simulink model "s0505_rollsensorfusion_CF"  (R2021a)
settings: Solver=FixedStepAuto  StartTime=0.0  StopTime=10.0  RelTol=1e-3  EnableMultiTasking=on
undefined symbols (not defined in the file or in its folder): Ts
libraries: CarMaker4SL x3, dspfdesign x1
settings Model: Creator=jason  LastModifiedBy=jason
settings ModelReferenceCC: ModelReferenceNumInstancesAllowed=Single

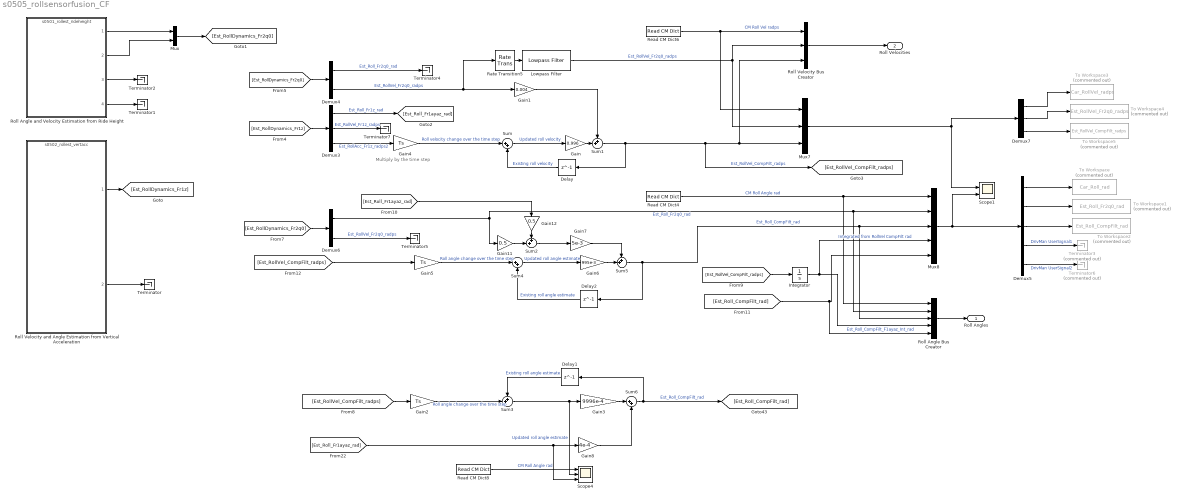
== system s0505_rollsensorfusion_CF ==
  note: Multiply by the time step
  Delay : Delay  DelayLength=1
  Delay1 : Delay  DelayLength=1
  Delay2 : Delay  DelayLength=1
  Demux3 : Demux  Outputs=3
      settings: DisplayOption=none
  Demux4 : Demux  Outputs=2
      settings: DisplayOption=none
  Demux5 : Demux  Outputs=5
      settings: DisplayOption=none
  Demux6 : Demux  Outputs=2
      settings: DisplayOption=none
  Demux7 : Demux  Outputs=3
  Gain : Gain  Gain=0.996
  Gain1 : Gain  Gain=0.004
  Gain11 : Gain  Gain=0.5
  Gain12 : Gain  Gain=0.5
  Gain2 : Gain  Gain=Ts
  Gain3 : Gain  Gain=9996e-4
  Gain4 : Gain  Gain=Ts
  Gain5 : Gain  Gain=Ts
  Gain6 : Gain  Gain=995e-3
  Gain7 : Gain  Gain=5e-3
  Gain8 : Gain  Gain=4e-4
  Integrator : Integrator
  Lowpass Filter : dspfdesign/Lowpass Filter  FilterType=FIR  DesignForMinimumOrder=on  FilterOrder=50  PassbandFrequency=1  StopbandFrequency=2000  PassbandRipple=0.1  StopbandAttenuation=180  InheritSampleRate=off  SampleRate=44100  SimulateUsing=Interpreted execution  roundingMode=Floor  coeffsDataTypeStr=fixdt(1,16)
  Mux : Mux  Inputs=2
  Mux7 : Mux  Inputs=3
  Mux8 : Mux  Inputs=5
  Rate Transition5 : RateTransition
  Read CM Dict4 : CarMaker4SL/Read CM Dict  xname=Car.Roll  xsync=off  xstime=Continuous
  Read CM Dict6 : CarMaker4SL/Read CM Dict  xname=Car.RollVel  xsync=off  xstime=Continuous
  Read CM Dict8 : CarMaker4SL/Read CM Dict  xname=Car.Roll  xsync=off  xstime=Continuous
  Roll Angle Bus Creator : BusCreator  Inputs=5  OutDataTypeStr=Bus: Est_Roll_CF
  Roll Angle and Velocity Estimation from Ride Height : ModelReference  ModelNameDialog=s0501_rollest_rideheight.slx  SimulationMode=Normal  ModelReferenceVersion=1.15
  Roll Velocity Bus Creator : BusCreator  Inputs=3  OutDataTypeStr=Bus: Est_RollVel_CF
  Roll Velocity and Angle Estimation from Vertical Acceleration : ModelReference  ModelNameDialog=s0502_rollest_vertacc.slx  SimulationMode=Normal  ModelReferenceVersion=1.17
  Scope1 : Scope  NumInputPorts=2
  Scope4 : Scope  NumInputPorts=3
  Sum : Sum  Inputs=|++
  Sum{1..3,5} (4 alike) : Sum  Inputs=++|
  Sum4 : Sum  Inputs=|++
  Sum6 : Sum  Inputs=|++
  Terminator{,1..2,4..5,7} (6 alike) : Terminator
  Terminator3 : Terminator  Commented=on
  Terminator6 : Terminator  Commented=on
  To Workspace : ToWorkspace  Commented=on  VariableName=Car_Roll_rad  SampleTime=-1
  To Workspace1 : ToWorkspace  Commented=on  VariableName=Est_Roll_Fr2q0_rad  SampleTime=-1
  To Workspace2 : ToWorkspace  Commented=on  VariableName=Est_Roll_CompFilt_rad  SampleTime=-1
  To Workspace3 : ToWorkspace  Commented=on  VariableName=Car_RollVel_radps  SampleTime=-1
  To Workspace4 : ToWorkspace  Commented=on  VariableName=Est_RollVel_Fr2q0_radps  SampleTime=-1
  To Workspace5 : ToWorkspace  Commented=on  VariableName=Est_RollVel_CompFilt_radps  SampleTime=-1
  Roll Angles : Outport  OutDataTypeStr=Bus: Est_Roll_CF
  Roll Velocities : Outport  Port=2  OutDataTypeStr=Bus: Est_RollVel_CF
  wires:
  Roll Angle and Velocity Estimation from Ride Height/2 -> Mux/2
  Roll Velocity and Angle Estimation from Vertical Acceleration/1 -> [Est_RollDynamics_Fr1z]
  Roll Angle and Velocity Estimation from Ride Height/1 -> Mux/1
  Roll Velocity and Angle Estimation from Vertical Acceleration/2 -> Terminator/1
  Roll Angle and Velocity Estimation from Ride Height/4 -> Terminator1/1
  Roll Angle and Velocity Estimation from Ride Height/3 -> Terminator2/1
  Mux/1 -> [Est_RollDynamics_Fr2q0]
  [Est_RollDynamics_Fr2q0] -> Demux4/1
  [Est_RollDynamics_Fr1z] -> Demux3/1
  Sum/1 -> Gain/1  "Updated roll velocity"
  Delay/1 -> Sum/2  "Existing roll velocity"
  Gain/1 -> Sum1/2
  Gain1/1 -> Sum1/1
  Demux4/2 -> Rate Transition5/1, Gain1/1  "Est_RollVel_Fr2q0_radps"
  Demux3/3 -> Gain4/1  "Est_RollAcc_Fr1z_radps2"
  Read CM Dict6/1 -> Mux7/1, Roll Velocity Bus Creator/1  "CM Roll Vel radps"
  Mux7/1 -> Demux7/1, Scope1/1
  Gain4/1 -> Sum/1  "Roll velocity change over the time step"
  Lowpass Filter/1 -> Mux7/2, Roll Velocity Bus Creator/2  "Est_RollVel_Fr2q0_radps"
  Rate Transition5/1 -> Lowpass Filter/1
  Demux3/1 -> [Est_Roll_Fr1ayaz_rad]  "Est_Roll_Fr1z_rad"
  Gain5/1 -> Sum4/1  "Roll angle change over the time step"
  Sum5/1 -> Roll Angle Bus Creator/3, Mux8/3, Delay2/1  "Est_Roll_CompFilt_rad"
  Delay2/1 -> Sum4/2  "Existing roll angle estimate"
  Gain6/1 -> Sum5/2
  Sum4/1 -> Gain6/1  "Updated roll angle estimate"
  [Est_RollDynamics_Fr2q0] -> Demux6/1
  Demux6/1 -> Gain11/1, Mux8/2, Roll Angle Bus Creator/2  "Est_Roll_Fr2q0_rad"
  Gain7/1 -> Sum5/1
  Demux4/1 -> Terminator4/1  "Est_Roll_Fr2q0_rad"
  Demux6/2 -> Terminator5/1  "Est_RollVel_Fr2q0_radps"
  Read CM Dict4/1 -> Mux8/1, Roll Angle Bus Creator/1  "CM Roll Angle rad"
  [Est_RollVel_CompFilt_radps] -> Gain5/1
  Sum3/1 -> Scope4/2, Gain3/1  "Updated roll angle estimate"
  Gain2/1 -> Sum3/2  "Roll angle change over the time step"
  Delay1/1 -> Sum3/1  "Existing roll angle estimate"
  Sum6/1 -> Delay1/1, [Est_Roll_CompFilt_rad]  "Est_Roll_CompFilt_rad"
  [Est_Roll_Fr1ayaz_rad] -> Scope4/3, Gain8/1
  Gain8/1 -> Sum6/2
  Gain3/1 -> Sum6/1
  [Est_RollVel_CompFilt_radps] -> Gain2/1
  Read CM Dict8/1 -> Scope4/1  "CM Roll Angle rad"
  [Est_RollVel_CompFilt_radps] -> Integrator/1
  Integrator/1 -> Mux8/4, Roll Angle Bus Creator/4  "Integrated from RollVel CompFilt rad"
  [Est_Roll_CompFilt_rad] -> Roll Angle Bus Creator/5, Mux8/5  "Est_Roll_CompFilt_F1ayaz_Int_rad"
  [Est_Roll_Fr1ayaz_rad] -> Gain12/1
  Gain11/1 -> Sum2/2
  Gain12/1 -> Sum2/1
  Sum2/1 -> Gain7/1
  Demux5/1 -> To Workspace/1
  Demux5/2 -> To Workspace1/1
  Demux5/3 -> To Workspace2/1
  Demux5/4 -> Terminator3/1  "DrivMan UserSignal1"
  Demux5/5 -> Terminator6/1  "DrivMan UserSignal2"
  Demux7/1 -> To Workspace3/1
  Demux7/2 -> To Workspace4/1
  Demux7/3 -> To Workspace5/1
  Sum1/1 -> Delay/1, Roll Velocity Bus Creator/3, Mux7/3, [Est_RollVel_CompFilt_radps]  "Est_RollVel_CompFilt_radps"
  Roll Velocity Bus Creator/1 -> Roll Velocities/1
  Roll Angle Bus Creator/1 -> Roll Angles/1
  Mux8/1 -> Demux5/1, Scope1/2
  Demux3/2 -> Terminator7/1  "Est_RollVel_Fr1z_radps"
